simulink model "hc_model"  (R2021b)
settings: Solver=VariableStepAuto  StartTime=0.0  StopTime=4  MaxStep=1e-3  RelTol=1e-3
values from neighbouring files (symbols this model uses):
  A = [zeros(4,4)      eye(4,4) ... (first row only)    [parameters.m]
  af = 0.8    [parameters.m]
  ar = 1.45    [parameters.m]
  B = [0 0 ... (first row only)    [parameters.m]
  C = [1 0 0 0 0 0 0 0 ... (first row only)    [parameters.m]
  c1 = 1500    [parameters.m]
  c2 = c1    (= 1500)    [parameters.m]
  D = [0 0 ... (first row only)    [parameters.m]
  Iyy = 600    [parameters.m]
  k1 = 21000    [parameters.m]
  k2 = k1    (= 21000)    [parameters.m]
  kt1 = 150000    [parameters.m]
  kt2 = kt1    (= 150000)    [parameters.m]
  m = 400    [parameters.m]
  m1 = 40    [parameters.m]
  m2 = m1    (= 40)    [parameters.m]
settings Model: Creator=maximesabbadini  LastModifiedBy=maximesabbadini

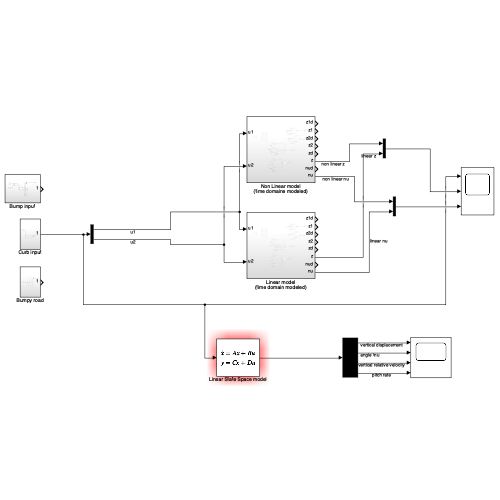
[thumbnail: Simulink's stored preview of the top-level diagram]
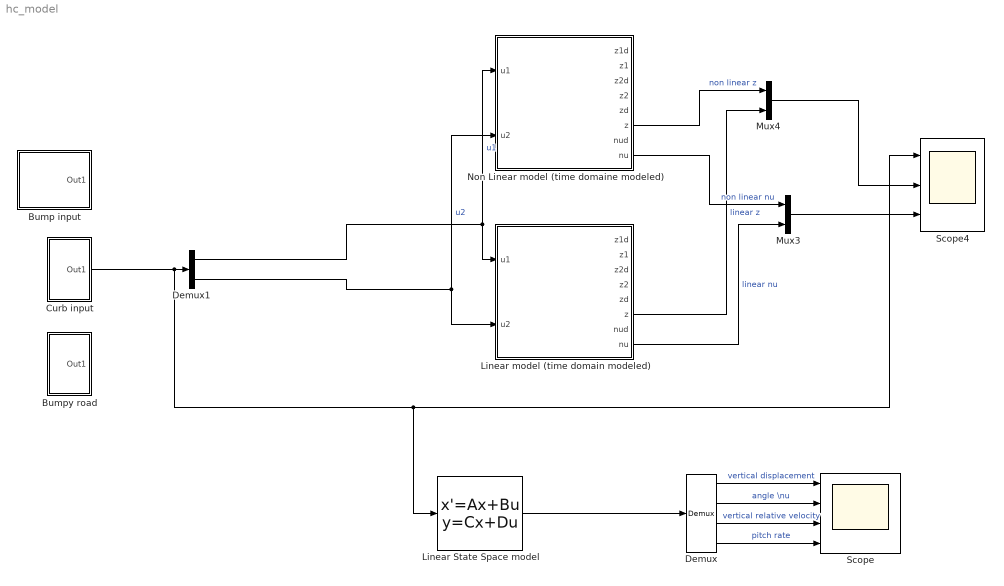
== system hc_model ==
  Bump input : Subsystem
  Bumpy road : Subsystem
  Curb input : Subsystem
  Demux : Demux
  Demux1 : Demux  Outputs=2
  Linear State Space model : StateSpace  A=A  B=B  C=C  D=D  InitialCondition=0
  Linear model (time domain modeled) : Subsystem
  Mux3 : Mux  Inputs=2
  Mux4 : Mux  Inputs=2
  Non Linear model (time domaine modeled) : Subsystem
  Scope : Scope  NumInputPorts=4
  Scope4 : Scope  NumInputPorts=3
  wires:
  Linear State Space model/1 -> Demux/1
  Non Linear model (time domaine modeled)/8(nu) -> Mux3/1  "non linear nu"
  Linear model (time domain modeled)/8(nu) -> Mux3/2  "linear nu"
  Mux3/1 -> Scope4/3
  Non Linear model (time domaine modeled)/6(z) -> Mux4/1  "non linear z"
  Linear model (time domain modeled)/6(z) -> Mux4/2  "linear z"
  Mux4/1 -> Scope4/2
  Curb input/1(Out1) -> Scope4/1, Linear State Space model/1, Demux1/1
  Demux1/1 -> Non Linear model (time domaine modeled)/1(u1), Linear model (time domain modeled)/1(u1)  "u1"
  Demux1/2 -> Non Linear model (time domaine modeled)/2(u2), Linear model (time domain modeled)/2(u2)  "u2"
  Demux/1 -> Scope/1  "vertical displacement"
  Demux/2 -> Scope/2  "angle \\nu"
  Demux/3 -> Scope/3  "vertical relative velocity"
  Demux/4 -> Scope/4  "pitch rate"

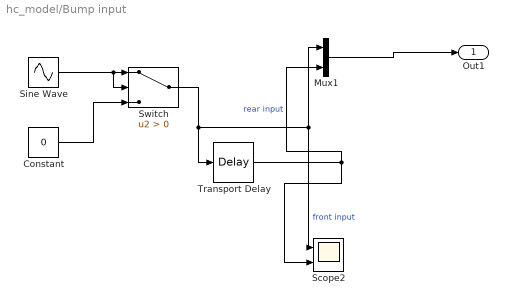
== system hc_model/Bump input ==
  Constant : Constant  Value=0
  Mux1 : Mux  Inputs=2
  Scope2 : Scope  NumInputPorts=2
  Sine Wave : Sin  Amplitude=.3  Frequency=1/2  SampleTime=0
  Switch : Switch  Criteria=u2 > Threshold
  Transport Delay : TransportDelay
  Out1 : Outport
  wires:
  Constant/1 -> Switch/3
  Mux1/1 -> Out1/1
  Sine Wave/1 -> Switch/2, Switch/1
  Switch/1 -> Transport Delay/1, Mux1/1, Scope2/1  "front input"
  Transport Delay/1 -> Mux1/2, Scope2/2  "rear input"

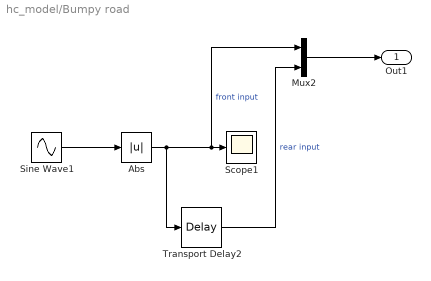
== system hc_model/Bumpy road ==
  Abs : Abs
  Mux2 : Mux  Inputs=2
  Scope1 : Scope
  Sine Wave1 : Sin  Amplitude=.05  Frequency=5  SampleTime=0
  Transport Delay2 : TransportDelay
  Out1 : Outport
  wires:
  Mux2/1 -> Out1/1
  Sine Wave1/1 -> Abs/1
  Abs/1 -> Transport Delay2/1, Mux2/1, Scope1/1  "front input"
  Transport Delay2/1 -> Mux2/2  "rear input"

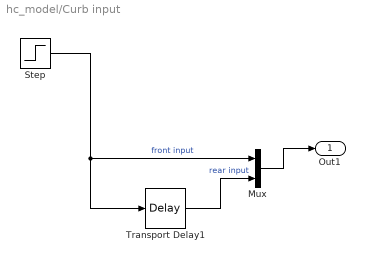
== system hc_model/Curb input ==
  Mux : Mux  Inputs=2
  Step : Step  After=.2  SampleTime=0
  Transport Delay1 : TransportDelay
  Out1 : Outport
  wires:
  Mux/1 -> Out1/1
  Step/1 -> Mux/1, Transport Delay1/1  "front input"
  Transport Delay1/1 -> Mux/2  "rear input"

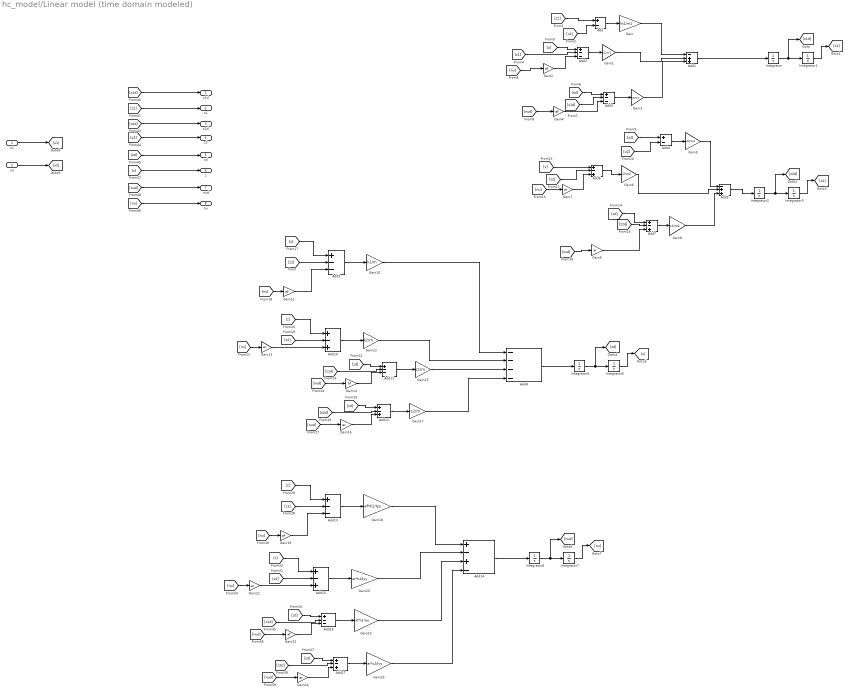
== system hc_model/Linear model (time domain modeled) ==
  u1 : Inport
  u2 : Inport  Port=2
  Add : Sum  Inputs=+-
  Add1 : Sum  Inputs=-++
  Add{6..7,10,12,15,17} (6 alike) : Sum  Inputs=+-+
  Add{2..3,9,11,13,16} (6 alike) : Sum  Inputs=+--
  Add14 : Sum  Inputs=+-+-
  Add4 : Sum  Inputs=+-
  Add5 : Sum  Inputs=-++
  Add8 : Sum  Inputs=----
  Gain : Gain  Gain=kt1/m1
  Gain1 : Gain  Gain=k1/m1
  Gain10 : Gain  Gain=k1/m
  Gain{2,4,11,14,19,22} (6 alike) : Gain  Gain=af
  Gain12 : Gain  Gain=k2/m
  Gain{7,9,13,16,21,24} (6 alike) : Gain  Gain=ar
  Gain15 : Gain  Gain=c1/m
  Gain17 : Gain  Gain=c2/m
  Gain18 : Gain  Gain=af*k1/Iyy
  Gain20 : Gain  Gain=ar*k2/Iyy
  Gain23 : Gain  Gain=af*c1/Iyy
  Gain25 : Gain  Gain=ar*c2/Iyy
  Gain3 : Gain  Gain=c1/m1
  Gain5 : Gain  Gain=kt2/m2
  Gain6 : Gain  Gain=k2/m2
  Gain8 : Gain  Gain=c2/m2
  Integrator{,1..7} (8 alike) : Integrator
  z1d : Outport
  z1 : Outport  Port=2
  z2d : Outport  Port=3
  z2 : Outport  Port=4
  zd : Outport  Port=5
  z : Outport  Port=6
  nud : Outport  Port=7
  nu : Outport  Port=8
  wires:
  Integrator/1 -> [z1d], Integrator1/1
  Integrator1/1 -> [z1]
  Integrator3/1 -> [z2]
  Integrator2/1 -> [z2d], Integrator3/1
  Integrator5/1 -> [z]
  Integrator4/1 -> [zd], Integrator5/1
  Integrator7/1 -> [nu]
  Integrator6/1 -> [nud], Integrator7/1
  u1/1 -> [u1]
  u2/1 -> [u2]
  [z1] -> Add/1
  [u1] -> Add/2
  Add/1 -> Gain/1
  Gain/1 -> Add1/1
  Gain1/1 -> Add1/2
  Add2/1 -> Gain1/1
  [z] -> Add2/1
  [z1] -> Add2/2
  [nu] -> Gain2/1
  Gain2/1 -> Add2/3
  Gain3/1 -> Add1/3
  Add3/1 -> Gain3/1
  [zd] -> Add3/1
  [z1d] -> Add3/2
  [nud] -> Gain4/1
  Gain4/1 -> Add3/3
  Add1/1 -> Integrator/1
  [u2] -> Add4/2
  [z2] -> Add4/1
  Add4/1 -> Gain5/1
  Gain5/1 -> Add5/1
  Add6/1 -> Gain6/1
  Gain6/1 -> Add5/2
  [z] -> Add6/1
  [z2] -> Add6/2
  [nu] -> Gain7/1
  Gain7/1 -> Add6/3
  Gain8/1 -> Add5/3
  Add7/1 -> Gain8/1
  [zd] -> Add7/1
  [z2d] -> Add7/2
  [nud] -> Gain9/1
  Gain9/1 -> Add7/3
  Add5/1 -> Integrator2/1
  Add9/1 -> Gain10/1
  [z] -> Add9/1
  [z1] -> Add9/2
  [nu] -> Gain11/1
  Gain11/1 -> Add9/3
  Gain10/1 -> Add8/1
  Add10/1 -> Gain12/1
  Gain13/1 -> Add10/3
  [z] -> Add10/1
  [nu] -> Gain13/1
  [z2] -> Add10/2
  Gain12/1 -> Add8/2
  [zd] -> Add11/1
  [z1d] -> Add11/2
  [nud] -> Gain14/1
  Gain14/1 -> Add11/3
  Add11/1 -> Gain15/1
  Gain15/1 -> Add8/3
  Gain16/1 -> Add12/3
  [nud] -> Gain16/1
  [zd] -> Add12/1
  Add12/1 -> Gain17/1
  [z2d] -> Add12/2
  Gain17/1 -> Add8/4
  Add8/1 -> Integrator4/1
  Gain19/1 -> Add13/3
  [z] -> Add13/1
  Add13/1 -> Gain18/1
  [z1] -> Add13/2
  [nu] -> Gain19/1
  Gain18/1 -> Add14/1
  [z] -> Add15/1
  [z2] -> Add15/2
  Add15/1 -> Gain20/1
  [nu] -> Gain21/1
  Gain21/1 -> Add15/3
  Gain20/1 -> Add14/2
  Gain22/1 -> Add16/3
  [nud] -> Gain22/1
  [zd] -> Add16/1
  Add16/1 -> Gain23/1
  [z1d] -> Add16/2
  Gain23/1 -> Add14/3
  [nud] -> Gain24/1
  Gain24/1 -> Add17/3
  [z2d] -> Add17/2
  Add17/1 -> Gain25/1
  [zd] -> Add17/1
  Gain25/1 -> Add14/4
  Add14/1 -> Integrator6/1
  [z1d] -> z1d/1
  [z1] -> z1/1
  [z2d] -> z2d/1
  [z2] -> z2/1
  [zd] -> zd/1
  [z] -> z/1
  [nud] -> nud/1
  [nu] -> nu/1

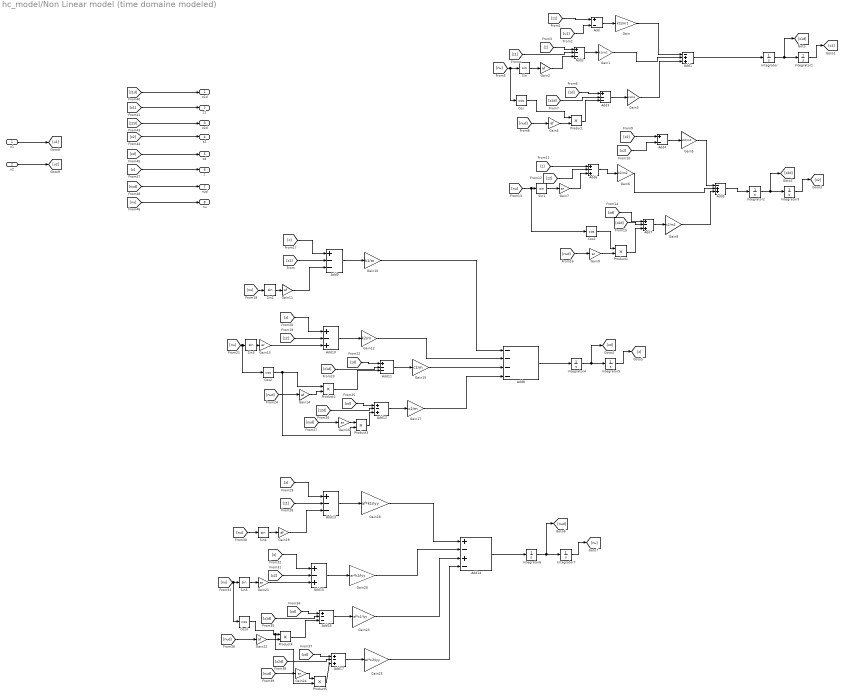
== system hc_model/Non Linear model (time domaine modeled) ==
  u1 : Inport
  u2 : Inport  Port=2
  Add : Sum  Inputs=+-
  Add1 : Sum  Inputs=-++
  Add{6..7,10,12,15,17} (6 alike) : Sum  Inputs=+-+
  Add{2..3,9,11,13,16} (6 alike) : Sum  Inputs=+--
  Add14 : Sum  Inputs=+-+-
  Add4 : Sum  Inputs=+-
  Add5 : Sum  Inputs=-++
  Add8 : Sum  Inputs=----
  Cos{,1..3} (4 alike) : Trigonometry  Operator=cos
  Gain : Gain  Gain=kt1/m1
  Gain1 : Gain  Gain=k1/m1
  Gain10 : Gain  Gain=k1/m
  Gain{2,4,11,14,19,22} (6 alike) : Gain  Gain=af
  Gain12 : Gain  Gain=k2/m
  Gain{7,9,13,16,21,24} (6 alike) : Gain  Gain=ar
  Gain15 : Gain  Gain=c1/m
  Gain17 : Gain  Gain=c2/m
  Gain18 : Gain  Gain=af*k1/Iyy
  Gain20 : Gain  Gain=ar*k2/Iyy
  Gain23 : Gain  Gain=af*c1/Iyy
  Gain25 : Gain  Gain=ar*c2/Iyy
  Gain3 : Gain  Gain=c1/m1
  Gain5 : Gain  Gain=kt2/m2
  Gain6 : Gain  Gain=k2/m2
  Gain8 : Gain  Gain=c2/m2
  Integrator{,1..7} (8 alike) : Integrator
  Product{,1..5} (6 alike) : Product
  Sin{,1..5} (6 alike) : Trigonometry
  z1d : Outport
  z1 : Outport  Port=2
  z2d : Outport  Port=3
  z2 : Outport  Port=4
  zd : Outport  Port=5
  z : Outport  Port=6
  nud : Outport  Port=7
  nu : Outport  Port=8
  wires:
  Integrator/1 -> [z1d], Integrator1/1
  Integrator1/1 -> [z1]
  Integrator3/1 -> [z2]
  Integrator2/1 -> [z2d], Integrator3/1
  Integrator5/1 -> [z]
  Integrator4/1 -> [zd], Integrator5/1
  Integrator7/1 -> [nu]
  Integrator6/1 -> [nud], Integrator7/1
  u1/1 -> [u1]
  u2/1 -> [u2]
  [z1] -> Add/1
  [u1] -> Add/2
  Add/1 -> Gain/1
  Gain/1 -> Add1/1
  Gain1/1 -> Add1/2
  Add2/1 -> Gain1/1
  [z] -> Add2/1
  [z1] -> Add2/2
  [nu] -> Cos/1, Sin/1
  Gain2/1 -> Add2/3
  Gain3/1 -> Add1/3
  Add3/1 -> Gain3/1
  [zd] -> Add3/1
  [z1d] -> Add3/2
  [nud] -> Gain4/1
  Add1/1 -> Integrator/1
  [u2] -> Add4/2
  [z2] -> Add4/1
  Add4/1 -> Gain5/1
  Gain5/1 -> Add5/1
  Add6/1 -> Gain6/1
  Gain6/1 -> Add5/2
  [z] -> Add6/1
  [z2] -> Add6/2
  [nu] -> Cos1/1, Sin1/1
  Gain7/1 -> Add6/3
  Gain8/1 -> Add5/3
  Add7/1 -> Gain8/1
  [zd] -> Add7/1
  [z2d] -> Add7/2
  [nud] -> Gain9/1
  Add5/1 -> Integrator2/1
  Add9/1 -> Gain10/1
  [z] -> Add9/1
  [z1] -> Add9/2
  [nu] -> Sin2/1
  Gain11/1 -> Add9/3
  Gain10/1 -> Add8/1
  Add10/1 -> Gain12/1
  Gain13/1 -> Add10/3
  [z] -> Add10/1
  [z2] -> Add10/2
  Gain12/1 -> Add8/2
  [zd] -> Add11/1
  [z1d] -> Add11/2
  [nud] -> Gain14/1
  Add11/1 -> Gain15/1
  Gain15/1 -> Add8/3
  [nud] -> Gain16/1
  [zd] -> Add12/1
  Add12/1 -> Gain17/1
  [z2d] -> Add12/2
  Gain17/1 -> Add8/4
  Add8/1 -> Integrator4/1
  Gain19/1 -> Add13/3
  [z] -> Add13/1
  Add13/1 -> Gain18/1
  [z1] -> Add13/2
  Gain18/1 -> Add14/1
  [z] -> Add15/1
  [z2] -> Add15/2
  Add15/1 -> Gain20/1
  Gain21/1 -> Add15/3
  Gain20/1 -> Add14/2
  [nud] -> Gain22/1
  [zd] -> Add16/1
  Add16/1 -> Gain23/1
  [z1d] -> Add16/2
  Gain23/1 -> Add14/3
  [nud] -> Gain24/1
  [z2d] -> Add17/2
  Add17/1 -> Gain25/1
  [zd] -> Add17/1
  Gain25/1 -> Add14/4
  Add14/1 -> Integrator6/1
  [z1d] -> z1d/1
  [z1] -> z1/1
  [z2d] -> z2d/1
  [z2] -> z2/1
  [zd] -> zd/1
  [z] -> z/1
  [nud] -> nud/1
  [nu] -> nu/1
  Sin/1 -> Gain2/1
  Gain4/1 -> Product/2
  Product/1 -> Add3/3
  Cos/1 -> Product/1
  Sin1/1 -> Gain7/1
  Product1/1 -> Add7/3
  Gain9/1 -> Product1/2
  Cos1/1 -> Product1/1
  Sin2/1 -> Gain11/1
  [nu] -> Cos2/1, Sin3/1
  Sin3/1 -> Gain13/1
  Gain14/1 -> Product2/2
  Cos2/1 -> Product3/2, Product2/1
  Product2/1 -> Add11/3
  Gain16/1 -> Product3/1
  Product3/1 -> Add12/3
  [nu] -> Sin4/1
  Sin4/1 -> Gain19/1
  [nu] -> Cos3/1, Sin5/1
  Sin5/1 -> Gain21/1
  Gain22/1 -> Product4/2
  Product4/1 -> Add16/3
  Cos3/1 -> Product5/2, Product4/1
  Gain24/1 -> Product5/1
  Product5/1 -> Add17/3
